simulink model "RiderPassThrough"  (R2025b)
settings: configuration reference "VehicleFixed1ms" (kept outside this file)
settings Model: DataDictionary=VirtualMotoTemplate.sldd  ModifiedByFormat=The MathWorks, Inc.  Creator=The MathWorks, Inc.  LastModifiedBy=The MathWorks, Inc.
settings ConfigSetRef: SourceName=VehicleFixed1ms

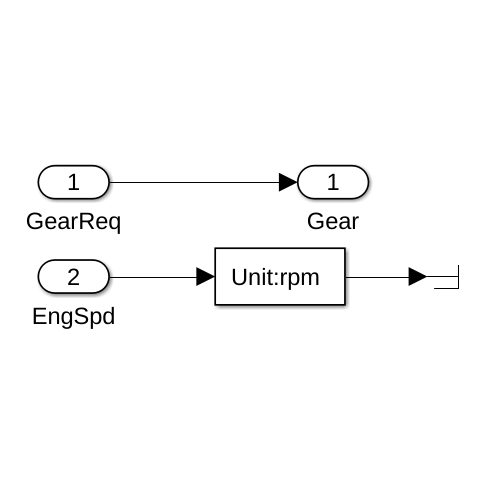
[thumbnail: Simulink's stored preview of the top-level diagram]
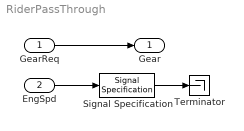
== system RiderPassThrough ==
  GearReq : Inport
  EngSpd : Inport  Port=2
  Signal Specification : SignalSpecification  Unit=rpm
  Terminator : Terminator
  Gear : Outport  VectorParamsAs1DForOutWhenUnconnected=off
  wires:
  GearReq/1 -> Gear/1
  EngSpd/1 -> Signal Specification/1
  Signal Specification/1 -> Terminator/1
